simulink model "hw2pendulumNL"  (R2013b)
settings: Solver=ode45  StartTime=0.0  StopTime=100  RelTol=1e-3
settings Model: Creator=czhang  LastModifiedBy=czhang

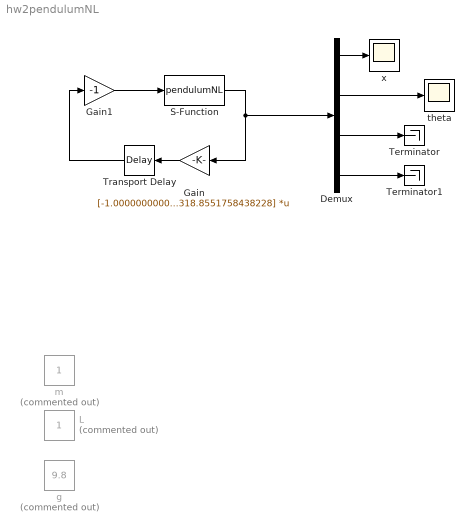
== system hw2pendulumNL ==
  Demux : Demux
  Gain : Gain  Gain="[-1.0000000000022 -325.6026451744055 -6.7416258738856  -318.8551758438228]"  Multiplication=Matrix(K*u)
  Gain1 : Gain  Gain=-1
  L : Constant  Commented=on
  S-Function : S-Function  FunctionName=pendulumNL  EnableBusSupport=off
  Terminator : Terminator
  Terminator1 : Terminator
  Transport Delay : TransportDelay  DelayTime=.28
  g : Constant  Commented=on  Value=9.8
  m : Constant  Commented=on
  theta : Scope
  x : Scope
  wires:
  Demux/4 -> Terminator1/1
  Demux/3 -> Terminator/1
  Demux/2 -> theta/1
  Demux/1 -> x/1
  Gain/1 -> Transport Delay/1
  Transport Delay/1 -> Gain1/1
  S-Function/1 -> Demux/1, Gain/1
  Gain1/1 -> S-Function/1
